simulink model "rtwdemo_logicOReml"  (Simulink 7.1)
settings: Solver=FixedStepDiscrete  StartTime=0.0  StopTime=10.0  RelTol=1e-3
settings Model: Creator=ajayaram  LastModifiedBy=ajayaram
settings OptimizationCC: OptimizeModelRefInitCode=on  LifeSpan=1
settings RTWCC: SystemTargetFile=ert.tlc  GenCodeOnly=on  GenerateMakefile=off  TemplateMakefile=ert_default_tmf  Description=Real-Time Workshop Embedded Coder (no auto configuration)  GenerateReport=on  ProcessScript=ert_make_rtw_hook  IncludeHyperlinkInReport=on  LaunchReport=on
settings CodeAppCC: GenerateComments=off  IgnoreCustomStorageClasses=off  SimulinkBlockComments=off
settings ERTTargetCC: GenerateSampleERTMain=on  InlinedParameterPlacement=NonHierarchical  ERTCustomFileTemplate=example_file_process.tlc

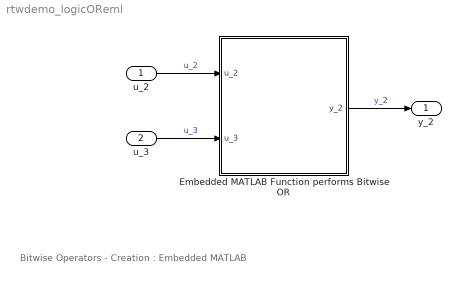
== system rtwdemo_logicOReml ==
  note: Bitwise Operators - Creation : Embedded MATLAB
  u_2 : Inport  DataType=uint8  OutDataType=sfix(16)  OutScaling=2^0  OutDataTypeStr=uint8
  u_3 : Inport  Port=2  DataType=uint8  OutDataType=sfix(16)  OutScaling=2^0  OutDataTypeStr=uint8
  Embedded MATLAB Function performs Bitwise OR : Stateflow chart
  y_2 : Outport  OutDataType=sfix(16)  OutScaling=2^0
  wires:
  u_2/1 -> Embedded MATLAB Function performs Bitwise OR/1(u_2)  "u_2"
  u_3/1 -> Embedded MATLAB Function performs Bitwise OR/2(u_3)  "u_3"
  Embedded MATLAB Function performs Bitwise OR/1(y_2) -> y_2/1  "y_2"

== matlab function Embedded MATLAB Function performs Bitwise OR ==
  data: u_2 input double; u_3 input double; y_2 output double
function y_2 = bitORer(u_2,u_3)

y_2 = bitor(u_2,u_3);
